simulink model "Motor_Pos_breach"  (R2017a)
settings: Solver=FixedStepAuto  StartTime=0.0  StopTime=tspan(end)  FixedStep=0.01  RelTol=1e-3
undefined symbols (not defined in the file or in its folder): b, J, K, L, R
settings Model: Creator=sansh  LastModifiedBy=nikhil
settings DataIOCC: ExternalInput=[t__, u__]  LoadExternalInput=on  SaveFormat=StructureWithTime  ReturnWorkspaceOutputs=on

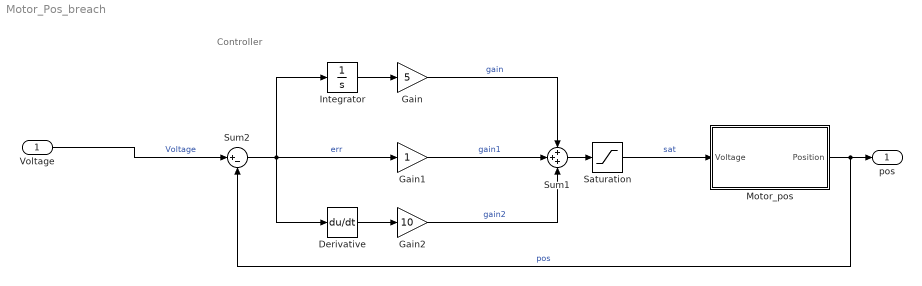
== system Motor_Pos_breach ==
  note: Controller
  Voltage : Inport
  Derivative : Derivative
  Gain : Gain  Gain=5
  Gain1 : Gain
  Gain2 : Gain  Gain=10
  Integrator : Integrator
  Motor_pos : Subsystem
  Saturation : Saturate  UpperLimit=10  LowerLimit=-10
  Sum1 : Sum  Inputs=+++
  Sum2 : Sum  Inputs=|+-
  pos : Outport
  wires:
  Motor_pos/1(Position) -> Sum2/2, pos/1  "pos"
  Sum1/1 -> Saturation/1
  Sum2/1 -> Derivative/1, Gain1/1, Integrator/1  "err"
  Voltage/1 -> Sum2/1  "Voltage"
  Gain2/1 -> Sum1/3  "gain2"
  Saturation/1 -> Motor_pos/1(Voltage)  "sat"
  Integrator/1 -> Gain/1
  Gain/1 -> Sum1/1  "gain"
  Derivative/1 -> Gain2/1
  Gain1/1 -> Sum1/2  "gain1"

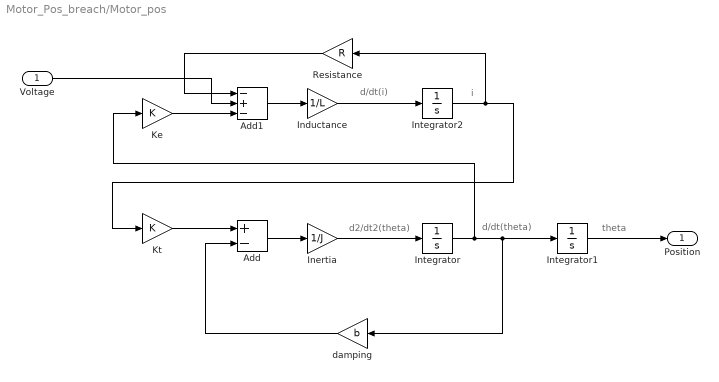
== system Motor_Pos_breach/Motor_pos ==
  note: i
  note: d/dt(i)
  note: d2/dt2(theta)
  note: d/dt(theta)
  note: theta
  Voltage : Inport
  Add : Sum  Inputs=+-
  Add1 : Sum  Inputs=-+-
  Inductance : Gain  Gain=1/L
  Inertia : Gain  Gain=1/J
  Integrator : Integrator
  Integrator1 : Integrator
  Integrator2 : Integrator
  Ke : Gain  Gain=K
  Kt : Gain  Gain=K
  Resistance : Gain  Gain=R
  damping : Gain  Gain=b
  Position : Outport
  wires:
  Inertia/1 -> Integrator/1
  Inductance/1 -> Integrator2/1
  Integrator2/1 -> Resistance/1, Kt/1
  Integrator/1 -> Ke/1, damping/1, Integrator1/1
  Integrator1/1 -> Position/1
  Voltage/1 -> Add1/2
  Add/1 -> Inertia/1
  damping/1 -> Add/2
  Kt/1 -> Add/1
  Resistance/1 -> Add1/1
  Ke/1 -> Add1/3
  Add1/1 -> Inductance/1
